simulink model "RPIDC"  (R2021a)
settings: Solver=ode45  StartTime=0.0  StopTime=SimulationTime  RelTol=1e-3  EnableMultiTasking=on
values from neighbouring files (symbols this model uses):
  c = 0    [RODPIDController.m]
  GCT = B*(1+(ea0^2)*(ro/E)*(wCT^2))    [RODPIDController.m]
  HCT = B*wCT^2    [RODPIDController.m]
  Kd = 3    [RODPIDController.m]
  Ki = 1.5    [RODPIDController.m]
  Kp = 5    [RODPIDController.m]
settings Model: Creator=Alireza  LastModifiedBy=Alireza
settings SolverCC: AlgebraicLoopSolver=TrustRegion
settings DataIOCC: LimitDataPoints=on  SaveFormat=Array  ReturnWorkspaceOutputs=off
settings OptimizationCC: LifeSpan=inf
settings DebuggingCC: SFUnexpectedBacktrackingDiag=warning  SFNoUnconditionalDefaultTransitionDiag=warning  SFExecutionAtInitializationDiag=none  SFMachineParentedDataDiag=warning  ArithmeticOperatorsInVariantConditions=warning
settings HardwareCC: ProdBitPerPointer=32  ProdBitPerSizeT=32  ProdBitPerPtrDiffT=32  ProdLargestAtomicFloat=None  ProdIntDivRoundTo=Undefined  ProdEndianess=Unspecified  ProdWordSize=32  ProdHWDeviceType=32-bit Generic
settings ModelReferenceCC: PropagateSignalLabelsOutOfModel=off
settings SFSimCC: SimUseLocalCustomCode=off  CustomCodeUndefinedFunction=UseInterfaceOnly
settings RTWCC: RTWUseLocalCustomCode=off
settings CodeAppCC: StateflowObjectComments=on
settings GRTTargetCC: TargetLangStandard=C89/C90 (ANSI)
settings ConfigComp: CovMetricSettings=dw  CovSaveCumulativeToWorkspaceVar=on  CovSaveSingleToWorkspaceVar=on  CovExternalEMLEnable=off

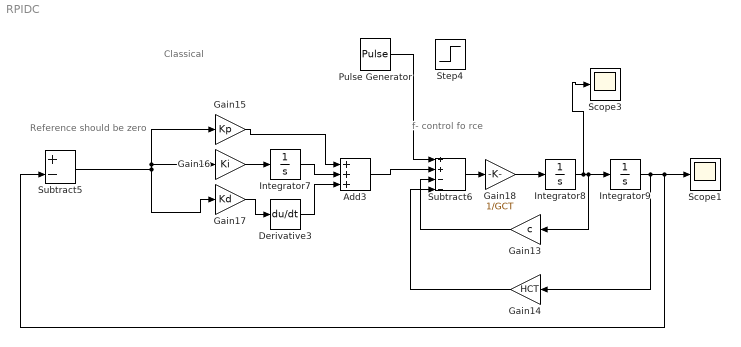
== system RPIDC ==
  note: Classical
  note: Reference should be zero
  note: f- control fo rce
  Add3 : Sum  Inputs=+++
  Derivative3 : Derivative
  Gain13 : Gain  Gain=c
  Gain14 : Gain  Gain=HCT
  Gain15 : Gain  Gain=Kp
  Gain16 : Gain  Gain=Ki
  Gain17 : Gain  Gain=Kd
  Gain18 : Gain  Gain=1/GCT
  Integrator7 : Integrator
  Integrator8 : Integrator
  Integrator9 : Integrator
  Pulse Generator : DiscretePulseGenerator  PulseType=Time based  Period=10
  Scope1 : Scope
  Scope3 : Scope
  Step4 : Step  SampleTime=0
  Subtract5 : Sum  Inputs=+-
  Subtract6 : Sum  Inputs=++--
  wires:
  Gain16/1 -> Integrator7/1
  Gain17/1 -> Derivative3/1
  Gain15/1 -> Add3/1
  Integrator7/1 -> Add3/2
  Derivative3/1 -> Add3/3
  Add3/1 -> Subtract6/2
  Subtract6/1 -> Gain18/1
  Gain18/1 -> Integrator8/1
  Integrator9/1 -> Subtract5/2, Scope1/1, Gain14/1
  Integrator8/1 -> Scope3/1, Gain13/1, Integrator9/1
  Gain13/1 -> Subtract6/3
  Gain14/1 -> Subtract6/4
  Subtract5/1 -> Gain15/1, Gain16/1, Gain17/1
  Pulse Generator/1 -> Subtract6/1
